simulink model "Monza_modelo"  (R2021b)
settings: Solver=VariableStepAuto  StartTime=0.0  StopTime=tsim  RelTol=1e-3
values from neighbouring files (symbols this model uses):
  dificultad = 1    [Modelin.m]
  v0 = 0.05    [Modelin.m]
  x0 = -0.11    [Modelin.m]
undefined symbols (not defined in the file or in its folder): mov_riel
settings Model: Creator=christian  LastModifiedBy=pablo
settings SolverCC: AlgebraicLoopSolver=TrustRegion
settings DataIOCC: ReturnWorkspaceOutputs=off
settings DebuggingCC: SFMachineParentedDataDiag=warning  ArithmeticOperatorsInVariantConditions=warning
settings SFSimCC: SimUseLocalCustomCode=off  CustomCodeUndefinedFunction=UseInterfaceOnly
settings RTWCC: RTWUseLocalCustomCode=off

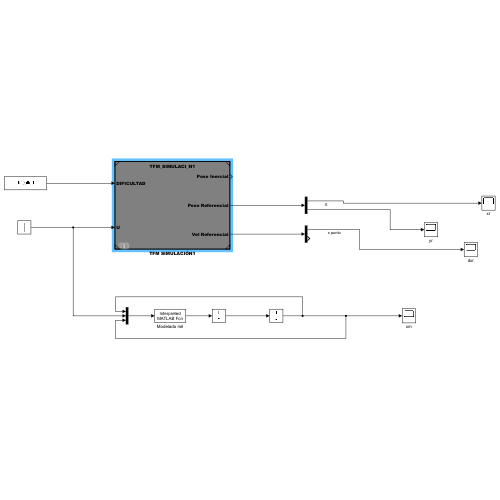
[thumbnail: Simulink's stored preview of the top-level diagram]
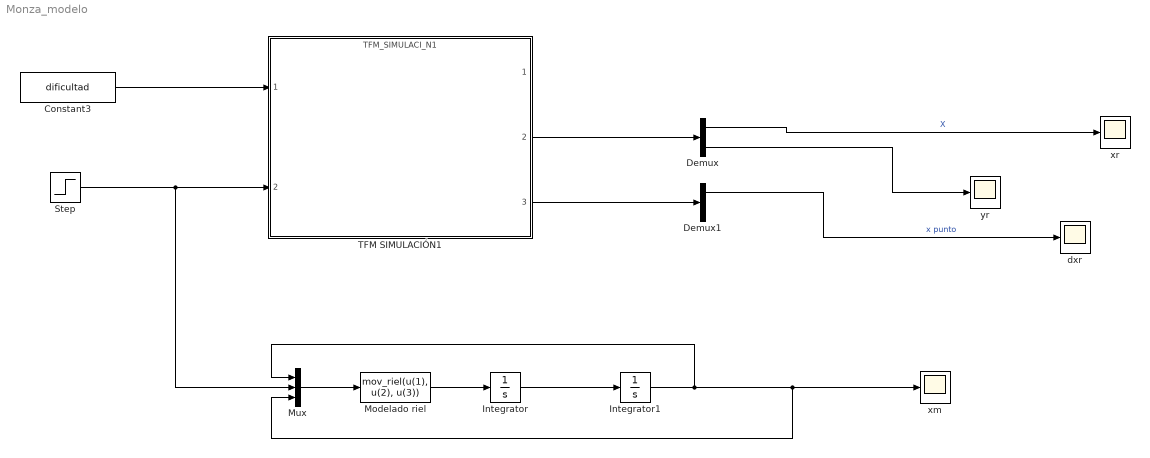
== system Monza_modelo ==
  Constant3 : Constant  Value=dificultad
  Demux : Demux  Outputs=2
  Demux1 : Demux  Outputs=2
  Integrator : Integrator  InitialCondition=v0
  Integrator1 : Integrator  InitialCondition=x0
  Modelado riel : MATLABFcn  MATLABFcn=mov_riel(u(1), u(2), u(3))
  Mux : Mux  Inputs=3
  Step : Step  Time=.2  Before=u  After=-.5  SampleTime=0
  TFM SIMULACIÓN1 : ModelReference  ModelNameDialog=TFM_SIMULACI_N1.slx  UsingDefaultArgumentValue=0,0  SimulationMode=Normal  ModelReferenceVersion=9.1  Gain=0.05  Gain2=0.0223  SimulationMode=Normal
  dxr : Scope
  xm : Scope
  xr : Scope
  yr : Scope
  wires:
  Constant3/1 -> TFM SIMULACIÓN1/1
  TFM SIMULACIÓN1/2 -> Demux/1
  TFM SIMULACIÓN1/3 -> Demux1/1
  Demux1/1 -> dxr/1  "x punto"
  Demux/1 -> xr/1  "X"
  Step/1 -> Mux/2, TFM SIMULACIÓN1/2
  Demux/2 -> yr/1
  Mux/1 -> Modelado riel/1
  Modelado riel/1 -> Integrator/1
  Integrator/1 -> Integrator1/1
  Integrator1/1 -> Mux/1, Mux/3, xm/1
